simulink model "ex2_7_sim"  (R2022b)
settings: Solver=VariableStepAuto  StartTime=0.0  StopTime=100  RelTol=1e-3
values from neighbouring files (symbols this model uses):
  Cth = Cp*m    (= 2042.03522483)    [ex2_7_cstes.m]
  Rconv = 1/(A*h)    (= 3.18309886184)    [ex2_6.m]    (also in ex2_7_cstes.m = 6.36619772368)
  Tinf = 240    [ex2_7_cstes.m]
  Tint = 1400    [ex2_7_cstes.m]
settings Model: Creator=nicol  LastModifiedBy=nicol

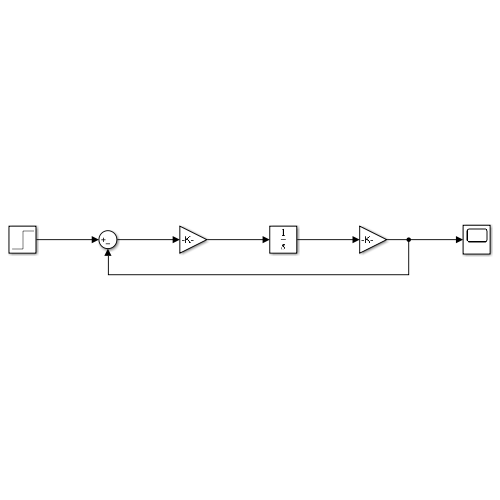
[thumbnail: Simulink's stored preview of the top-level diagram]
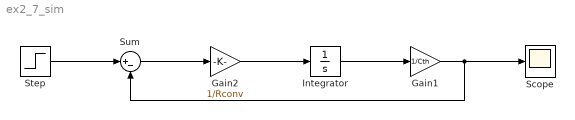
== system ex2_7_sim ==
  Gain1 : Gain  Gain=1/Cth
  Gain2 : Gain  Gain=1/Rconv
  Integrator : Integrator  InitialCondition=Tint*Cth
  Scope : Scope
  Step : Step  Time=0  After=Tinf  SampleTime=0
  Sum : Sum  Inputs=|+-
  wires:
  Integrator/1 -> Gain1/1
  Gain2/1 -> Integrator/1
  Sum/1 -> Gain2/1
  Gain1/1 -> Sum/2, Scope/1
  Step/1 -> Sum/1
